simulink model "float_sch_Sample_HardThreshold"  (R2020a)
settings: Solver=VariableStepAuto  StartTime=0  StopTime=60  RelTol=1e-3
model workspace (MAT data in the model file):
  a = 0
values from neighbouring files (symbols this model uses):
  fs = 30000    [float_sch_run_LocalMaxima_AdaptiveThreshold.m]    (also in float_sch_run_LocalMaxima_HardThreshold.m; float_sch_run_PTSD.m; float_sch_run_Sample_AdaptiveThreshold.m; float_sch_run_Sample_HardThreshold.m)
  refractory = 10^-3    (= 0.001)    [float_sch_run_LocalMaxima_AdaptiveThreshold.m]    (also in float_sch_run_LocalMaxima_HardThreshold.m; float_sch_run_PTSD.m; float_sch_run_Sample_AdaptiveThreshold.m; float_sch_run_Sample_HardThreshold.m)
  th = [-60]    [float_sch_run_LocalMaxima_HardThreshold.m]    (also in float_sch_run_Sample_HardThreshold.m = [-75:1:-25])
libraries: dspfdesign x2, simulink x2, dspswit3 x1, hdlsllib x1
settings Model: SimulationMode=rapid-accelerator  Creator=sbuccelli  LastModifiedBy=diflo
settings DebuggingCC: SignalRangeChecking=warning

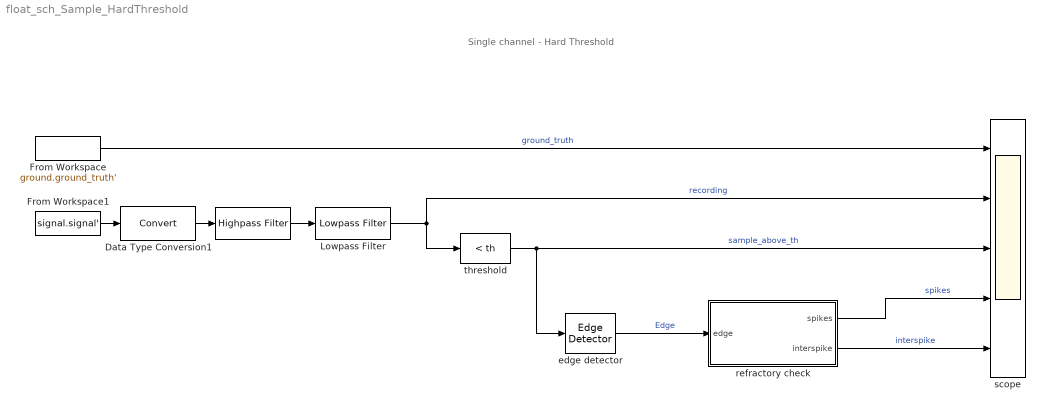
== system float_sch_Sample_HardThreshold ==
  note: Single channel - Hard Threshold
  " " : dspfdesign/Highpass Filter  FilterType=IIR  DesignForMinimumOrder=on  FilterOrder=50  StopbandFrequency=1  PassbandFrequency=300  StopbandAttenuation=80  PassbandRipple=0.1  InheritSampleRate=off  SampleRate=fs  SimulateUsing=Interpreted execution  roundingMode=Floor  coeffsDataTypeStr=fixdt(1,16)
  Data Type Conversion1 : DataTypeConversion
  From Workspace : FromWorkspace  VariableName=ground.ground_truth'  SampleTime=1/fs
  From Workspace1 : FromWorkspace  VariableName=signal.signal'  SampleTime=1/fs
  Lowpass Filter : dspfdesign/Lowpass Filter  FilterType=IIR  DesignForMinimumOrder=on  FilterOrder=3  PassbandFrequency=3500  StopbandFrequency=8500  PassbandRipple=0.1  StopbandAttenuation=80  InheritSampleRate=off  SampleRate=fs  SimulateUsing=Interpreted execution  roundingMode=Floor  coeffsDataTypeStr=fixdt(1,16)
  "edge detector " : dspswit3/Edge Detector  InputProcessing=Columns as channels (frame based)
      settings: SourceProductBaseCode=DS
  refractory check : Subsystem
  scope : Scope  NumInputPorts=5
  threshold : simulink/Logic and Bit Operations/Compare To Constant  relop=<  const=th  OutDataTypeStr=boolean
  wires:
  threshold/1 -> scope/3, "edge detector "/1  "sample_above_th"
  From Workspace1/1 -> Data Type Conversion1/1
  "edge detector "/1 -> refractory check/1("edge  ")  "Edge"
  refractory check/2(interspike) -> scope/5  "interspike"
  refractory check/1(spikes) -> scope/4  "spikes"
  " "/1 -> Lowpass Filter/1
  Lowpass Filter/1 -> threshold/1, scope/2  "recording"
  From Workspace/1 -> scope/1  "ground_truth"
  Data Type Conversion1/1 -> " "/1

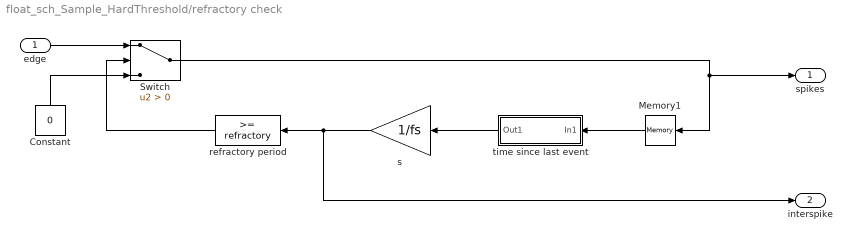
== system float_sch_Sample_HardThreshold/refractory check ==
  "edge  " : Inport
  Constant : Constant  Value=0
  Memory1 : Memory  InheritSampleTime=on
  Switch : Switch  Criteria=u2 > Threshold
  refractory period : simulink/Logic and Bit Operations/Compare To Constant  relop=>=  const=refractory  OutDataTypeStr=boolean
  s : Gain  Gain=1/fs  ParamDataTypeStr=double
  time since last event : Subsystem
  spikes : Outport
  interspike : Outport  Port=2
  wires:
  "edge  "/1 -> Switch/1
  Memory1/1 -> time since last event/1(In1)
  time since last event/1(Out1) -> s/1
  Constant/1 -> Switch/3
  s/1 -> refractory period/1, interspike/1
  Switch/1 -> spikes/1, Memory1/1
  refractory period/1 -> Switch/2

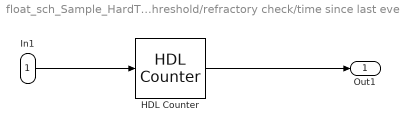
== system float_sch_Sample_HardThreshold/refractory check/time since last event ==
  In1 : Inport
  HDL Counter : hdlsllib/Sources/HDL Counter  CountType=Free running  CountInit=1  CountStep=1  CountMax=25  CountFromType=Initial value  CountFrom=1  CountResetPort=on  CountLoadPort=off  CountEnbPort=off  CountDirPort=off  CountDataType=Unsigned  CountWordLen=16  CountFracLen=0  CountSampTime=1
  Out1 : Outport
  wires:
  In1/1 -> HDL Counter/1
  HDL Counter/1 -> Out1/1
